simulink model "BirdEyeView_Bilinear_V1"  (R2022a)
settings: Solver=FixedStepDiscrete  StartTime=0.0  StopTime=Ts_480p*4  RelTol=1e-3
InitFcn:
  | Ts = 1e-3;
  | Ts_240p = 402*324*Ts;
  | Ts_480p = 525*800*Ts;
  | %global lut;
  | %temp = load('lut_rc_c.mat');
  | %lut = temp.lut_rc_c;
undefined symbols (not defined in the file or in its folder): gray, Rec, SDTV
libraries: hdlsllib x13, visionhdlio x2, visionhdlconversions x1, dspvision x1
settings Model: DataTypeOverride=Off  ModifiedByFormat=4mbilal@gmail.com  Creator=The MathWorks, Inc.  LastModifiedBy=4mbilal@gmail.com
settings SolverCC: AlgebraicLoopSolver=TrustRegion
settings DataIOCC: LimitDataPoints=on  SaveFormat=Array  SaveOutput=off  SaveTime=off  ReturnWorkspaceOutputs=off
settings OptimizationCC: BlockReduction=off  ConditionallyExecuteInputs=off  DefaultParameterBehavior=Inlined  LifeSpan=inf
settings DebuggingCC: AlgebraicLoopMsg=error  SolverPrmCheckMsg=warning  SingleTaskRateTransMsg=error  ParameterPrecisionLossMsg=none  UnconnectedInputMsg=warning  UnconnectedOutputMsg=warning  UnconnectedLineMsg=warning  AllowSymbolicDim=off  SFUnexpectedBacktrackingDiag=warning  SFNoUnconditionalDefaultTransitionDiag=warning  SFExecutionAtInitializationDiag=none  SFMachineParentedDataDiag=warning  IntegerSaturationMsg=none  ArithmeticOperatorsInVariantConditions=warning
settings HardwareCC: ProdBitPerPointer=32  ProdBitPerSizeT=32  ProdBitPerPtrDiffT=32  ProdLargestAtomicFloat=None  ProdIntDivRoundTo=Undefined  ProdEndianess=Unspecified  ProdWordSize=32  ProdHWDeviceType=ASIC/FPGA->ASIC/FPGA  ProdEqTarget=off
settings ModelReferenceCC: PropagateSignalLabelsOutOfModel=off
settings SFSimCC: SimUseLocalCustomCode=off  CustomCodeUndefinedFunction=UseInterfaceOnly
settings RTWCC: RTWUseLocalCustomCode=off
settings CodeAppCC: StateflowObjectComments=on
settings GRTTargetCC: TargetLangStandard=C89/C90 (ANSI)
settings ConfigComp: CovMetricSettings=dw  CovSaveCumulativeToWorkspaceVar=on  CovSaveSingleToWorkspaceVar=on  CovExternalEMLEnable=off  CovSFcnEnable=off

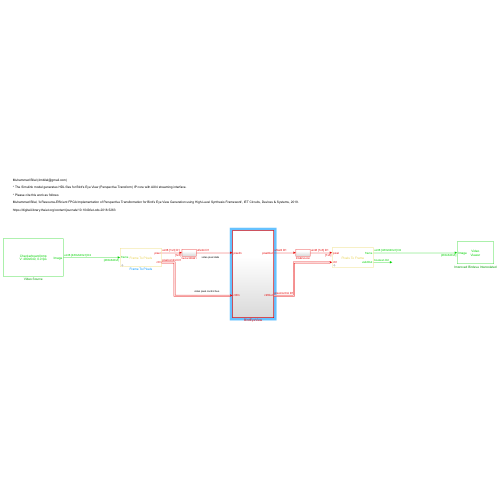
[thumbnail: Simulink's stored preview of the top-level diagram]
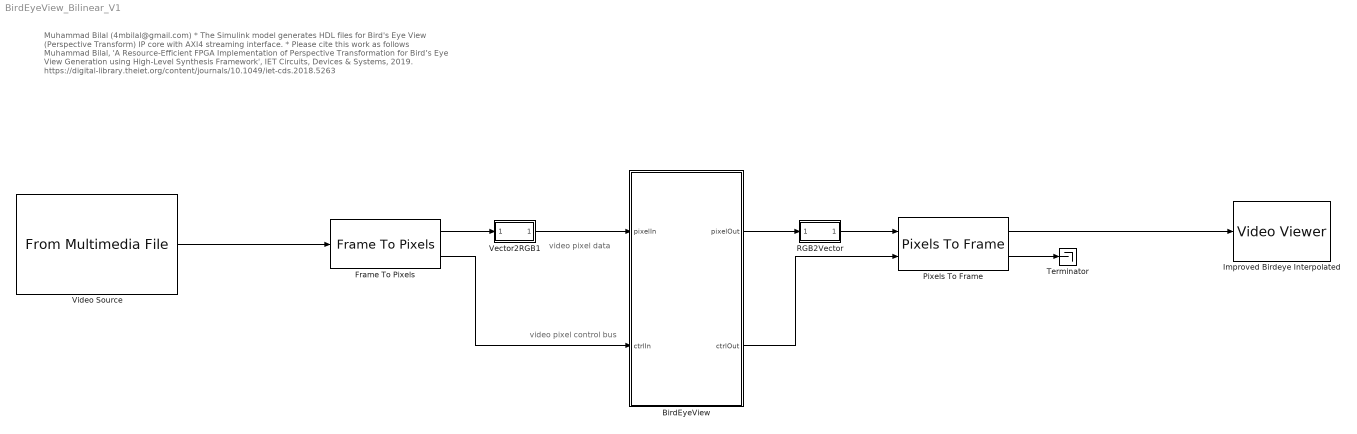
== system BirdEyeView_Bilinear_V1 ==
  note: Muhammad Bilal (4mbilal@gmail.com)
      |
      | * The Simulink model generates HDL files for Bird's Eye View (Perspective Transform) IP core with AXI4 streaming interface.
      |
      | * Please cite this work as follows
      |
      | Muhammad Bilal, 'A Resource-Efficient FPGA Implementation of Perspective Transformation for Bird’s Eye View Generation using High-Level Synthesis Framework', IET Circuits, Devices & Systems, 2019.
      |
      | https://digital-library.theiet.org/content/journals/10.1049/iet-cds.2018.5263
  note: video pixel data
  note: video pixel control bus
  BirdEyeView : Subsystem  TreatAsAtomicUnit=on
  Frame To Pixels : visionhdlio/Frame To Pixels  NumComponents=3  NumPixels=1  VideoFormat=480p  ActivePixelsPerLine=640  ActiveVideoLines=480  TotalPixelsPerLine=800  TotalVideoLines=525  StartingActiveLine=36  FrontPorch=16  SampleTime=0  VideoFormatCache=480p  ActivePixelsPerLineCache=32  ActiveVideoLinesCache=18  TotalPixelsPerLineCache=42  TotalVideoLinesCache=28  StartingActiveLineCache=6  FrontPorchCache=5
      settings: SourceProductBaseCode=VT
  Improved Birdeye Interpolated : VideoViewer  colormapValue=gray(256)  FigPos=[601 632.4 660.8 447.2]
  Pixels To Frame : visionhdlio/Pixels To Frame  NumComponents=3  NumPixels=1  VideoFormat=480p  ActivePixelsPerLine=640  ActiveVideoLines=480  TotalPixelsPerLine=800  TotalVideoLines=525  VideoFormatCache=480p  ActivePixelsPerLineCache=32  ActiveVideoLinesCache=18  TotalPixelsPerLineCache=42  TotalVideoLinesCache=28
      settings: SourceProductBaseCode=VT
  RGB2Vector : Subsystem
  Terminator : Terminator
  Vector2RGB1 : Subsystem
  Video Source : dspvision/From Multimedia File  inputFilename=D:\Zedboard\custom_ip_cores\Mathworks\BirdsEyeView\Checkerboard.bmp  readRange=[1 Inf]  loop=on  numPlays=inf  outputStreams=Video only  videoDataType=uint8  audioDataType=int16  inheritSampleTime=off  userDefinedSampleTime=Ts_480p  noAudioOutput=off  isIntensityVideo=off  fourcc=RGB  colorVideoFormat=One multidimensional signal  outputEOF=off  dataOrg=Column-major  audioFrameSize=1024  computeAudioFrameSize=off  outSamplingMode=Sample based
  wires:
  Pixels To Frame/2 -> Terminator/1
  Vector2RGB1/1(RGB) -> BirdEyeView/1(pixelIn)
  BirdEyeView/1(pixelOut) -> RGB2Vector/1(RGB)
  Frame To Pixels/1 -> Vector2RGB1/1(RGBVector)
  BirdEyeView/2(ctrlOut) -> Pixels To Frame/2
  Frame To Pixels/2 -> BirdEyeView/2(ctrlIn)
  RGB2Vector/1(RGBVector) -> Pixels To Frame/1
  Pixels To Frame/1 -> Improved Birdeye Interpolated/1
  Video Source/1 -> Frame To Pixels/1

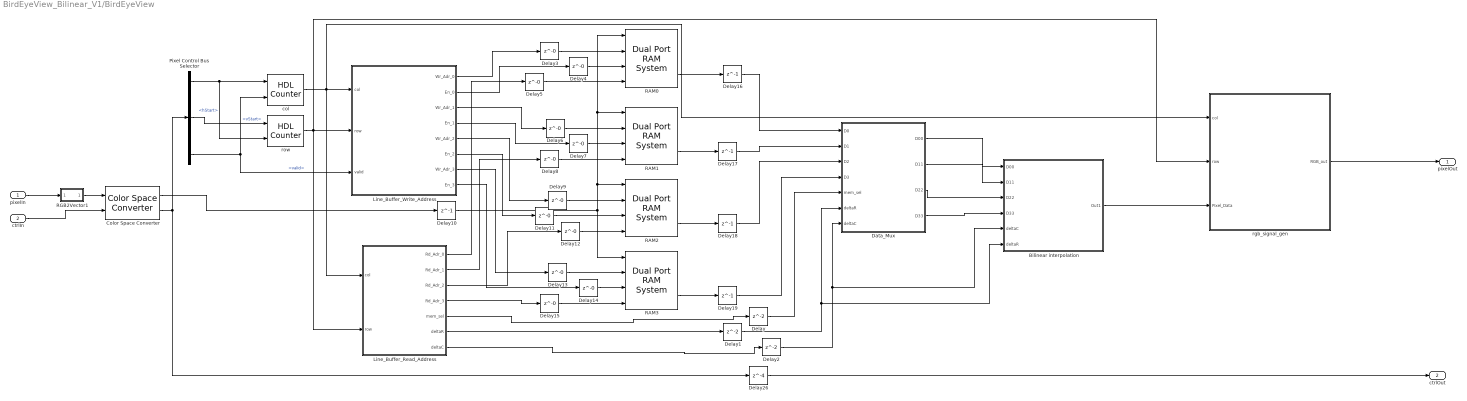
== system BirdEyeView_Bilinear_V1/BirdEyeView ==
  pixelIn : Inport
  ctrlIn : Inport  Port=2
  Bilinear interpolation : Subsystem
  Color Space Converter : visionhdlconversions/Color Space Converter  Conversion=RGB to intensity  ConversionStandard=Rec. 601 (SDTV)  ScanningStandard=1250/50/2:1  SimulateUsing=Code generation
      settings: SourceProductBaseCode=VT
  Data_Mux : MATLAB Function  TreatAsAtomicUnit=on
  Delay : Delay  InitialCondition=0
  Delay1 : Delay  InitialCondition=0
  Delay{10,16..19} (5 alike) : Delay  DelayLength=1  InitialCondition=0
  Delay{3..9,11..15} (12 alike) : Delay  DelayLength=0  InitialCondition=0
  Delay2 : Delay  InitialCondition=0
  Delay26 : Delay  DelayLength=4  InitialCondition=0
  Line_Buffer_Read_Address : MATLAB Function  TreatAsAtomicUnit=on
  Line_Buffer_Write_Address : MATLAB Function  TreatAsAtomicUnit=on
  Pixel Control Bus Selector : BusSelector  OutputSignals=hStart,hEnd,vStart,vEnd,valid
  RAM{0..3} (4 alike) : hdlsllib/HDL RAMs/Dual Port RAM System  RAMType=Dual port  WriteOutputValue=New data  RAMInitialValue=0  SimulateUsing=Code generation
      settings: SourceProductBaseCode=SL
  RGB2Vector1 : Subsystem
  col : hdlsllib/Sources/HDL Counter  CountType=Count limited  CountInit=0  CountStep=1  CountMax=638  CountFromType=Initial value  CountFrom=0  CountResetPort=on  CountLoadPort=off  CountEnbPort=on  CountDirPort=off  CountHitOutputPort=off  CountDataType=Unsigned  CountWordLen=10  CountFracLen=0  CountSampTime=1
  rgb_signal_gen : MATLAB Function  TreatAsAtomicUnit=on
  row : hdlsllib/Sources/HDL Counter  CountType=Count limited  CountInit=0  CountStep=1  CountMax=638  CountFromType=Initial value  CountFrom=0  CountResetPort=on  CountLoadPort=off  CountEnbPort=on  CountDirPort=off  CountHitOutputPort=off  CountDataType=Unsigned  CountWordLen=10  CountFracLen=0  CountSampTime=1
  pixelOut : Outport  VectorParamsAs1DForOutWhenUnconnected=off
  ctrlOut : Outport  Port=2  VectorParamsAs1DForOutWhenUnconnected=off
  wires:
  ctrlIn/1 -> Color Space Converter/2
  pixelIn/1 -> RGB2Vector1/1(RGB)
  RGB2Vector1/1(RGBVector) -> Color Space Converter/1
  rgb_signal_gen/1(RGB_out) -> pixelOut/1
  Color Space Converter/2 -> Delay26/1, Pixel Control Bus Selector/1
  Pixel Control Bus Selector/1 -> row/2, col/1  "<hStart>"
  col/1 -> Line_Buffer_Read_Address/1(col), Line_Buffer_Write_Address/1(col), rgb_signal_gen/1(col)
  Pixel Control Bus Selector/5 -> Line_Buffer_Write_Address/3(valid), col/2  "<valid>"
  Pixel Control Bus Selector/3 -> row/1  "<vStart>"
  row/1 -> Line_Buffer_Read_Address/2(row), Line_Buffer_Write_Address/2(row), rgb_signal_gen/2(row)
  Color Space Converter/1 -> Delay10/1
  Line_Buffer_Write_Address/1(Wr_Adr_0) -> Delay3/1
  Line_Buffer_Write_Address/2(En_0) -> Delay4/1
  Line_Buffer_Write_Address/3(Wr_Adr_1) -> Delay6/1
  Line_Buffer_Write_Address/4(En_1) -> Delay7/1
  Line_Buffer_Write_Address/5(Wr_Adr_2) -> Delay9/1
  Line_Buffer_Write_Address/6(En_2) -> Delay11/1
  Line_Buffer_Write_Address/7(Wr_Adr_3) -> Delay13/1
  Line_Buffer_Write_Address/8(En_3) -> Delay14/1
  Line_Buffer_Read_Address/1(Rd_Adr_0) -> Delay5/1
  Line_Buffer_Read_Address/2(Rd_Adr_1) -> Delay8/1
  Line_Buffer_Read_Address/3(Rd_Adr_2) -> Delay12/1
  Line_Buffer_Read_Address/4(Rd_Adr_3) -> Delay15/1
  RAM0/2 -> Delay16/1
  RAM1/2 -> Delay17/1
  RAM2/2 -> Delay18/1
  RAM3/2 -> Delay19/1
  Line_Buffer_Read_Address/5(mem_sel) -> Delay/1
  Line_Buffer_Read_Address/6(deltaR) -> Delay1/1
  Line_Buffer_Read_Address/7(deltaC) -> Delay2/1
  Delay/1 -> Data_Mux/5(mem_sel)
  Delay1/1 -> Data_Mux/6(deltaR), Bilinear interpolation/6(deltaR)
  Delay2/1 -> Data_Mux/7(deltaC), Bilinear interpolation/5(deltaC)
  Delay3/1 -> RAM0/2
  Delay4/1 -> RAM0/3
  Delay5/1 -> RAM0/4
  Delay6/1 -> RAM1/2
  Delay7/1 -> RAM1/3
  Delay8/1 -> RAM1/4
  Delay9/1 -> RAM2/2
  Delay10/1 -> RAM0/1, RAM1/1, RAM2/1, RAM3/1
  Delay11/1 -> RAM2/3
  Delay12/1 -> RAM2/4
  Delay13/1 -> RAM3/2
  Delay14/1 -> RAM3/3
  Delay15/1 -> RAM3/4
  Delay16/1 -> Data_Mux/1(D0)
  Delay17/1 -> Data_Mux/2(D1)
  Delay18/1 -> Data_Mux/3(D2)
  Delay19/1 -> Data_Mux/4(D3)
  Delay26/1 -> ctrlOut/1
  Data_Mux/1(D00) -> Bilinear interpolation/1(D00)
  Data_Mux/2(D11) -> Bilinear interpolation/2(D11)
  Data_Mux/3(D22) -> Bilinear interpolation/3(D22)
  Data_Mux/4(D33) -> Bilinear interpolation/4(D33)
  Bilinear interpolation/1(Out1) -> rgb_signal_gen/3(Pixel_Data)

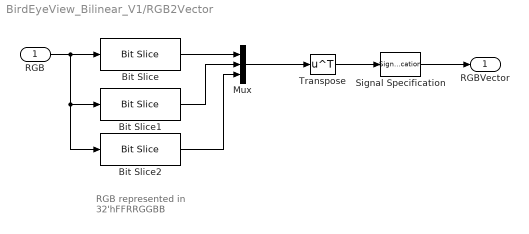
== system BirdEyeView_Bilinear_V1/RGB2Vector ==
  note: RGB represented in
      | 32'hFFRRGGBB
  RGB : Inport
  Bit Slice : hdlsllib/Logic and Bit Operations/Bit Slice  lidx=23  ridx=16
      settings: SourceProductBaseCode=SL
  Bit Slice1 : hdlsllib/Logic and Bit Operations/Bit Slice  lidx=15  ridx=8
      settings: SourceProductBaseCode=SL
  Bit Slice2 : hdlsllib/Logic and Bit Operations/Bit Slice  lidx=7  ridx=0
      settings: SourceProductBaseCode=SL
  Mux : Mux  Inputs=3
  Signal Specification : SignalSpecification
  Transpose : Math  Operator=transpose  SignedPower=on
  RGBVector : Outport  VectorParamsAs1DForOutWhenUnconnected=off
  wires:
  Mux/1 -> Transpose/1
  Bit Slice/1 -> Mux/1
  Bit Slice2/1 -> Mux/3
  Bit Slice1/1 -> Mux/2
  RGB/1 -> Bit Slice2/1, Bit Slice1/1, Bit Slice/1
  Transpose/1 -> Signal Specification/1
  Signal Specification/1 -> RGBVector/1

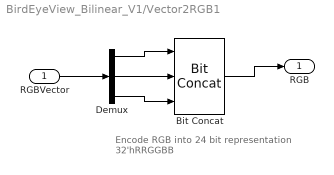
== system BirdEyeView_Bilinear_V1/Vector2RGB1 ==
  note: Encode RGB into 24 bit representation
      | 32'hRRGGBB
  RGBVector : Inport
  Bit Concat : hdlsllib/Logic and Bit Operations/Bit Concat  numInputs=3
  Demux : Demux  Outputs=3
  RGB : Outport  VectorParamsAs1DForOutWhenUnconnected=off
  wires:
  Bit Concat/1 -> RGB/1
  RGBVector/1 -> Demux/1
  Demux/1 -> Bit Concat/1
  Demux/2 -> Bit Concat/2
  Demux/3 -> Bit Concat/3

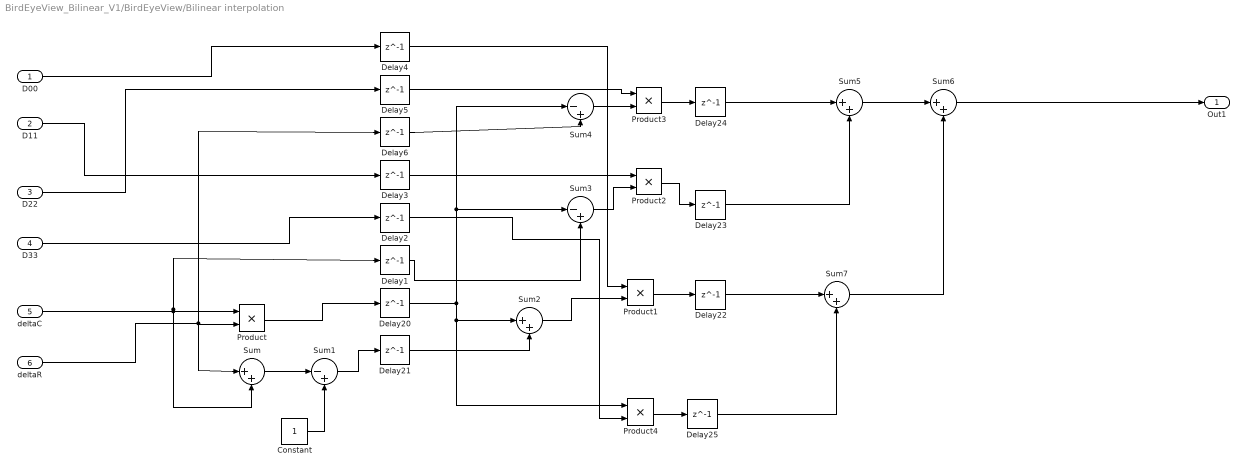
== system BirdEyeView_Bilinear_V1/BirdEyeView/Bilinear interpolation ==
  D00 : Inport
  D11 : Inport  Port=2
  D22 : Inport  Port=3
  D33 : Inport  Port=4
  deltaC : Inport  Port=5
  deltaR : Inport  Port=6
  Constant : Constant  OutDataTypeStr=boolean
  Delay{1..6,20..25} (12 alike) : Delay  DelayLength=1  InitialCondition=0
  Product{,1..4} (5 alike) : Product
  Sum{,2,5..7} (5 alike) : Sum  Inputs=|++
  Sum1 : Sum  Inputs=|-+
  Sum3 : Sum  Inputs=|-+
  Sum4 : Sum  Inputs=|-+
  Out1 : Outport  VectorParamsAs1DForOutWhenUnconnected=off
  wires:
  D11/1 -> Delay3/1
  Product1/1 -> Delay22/1
  Sum4/1 -> Product3/2
  Product3/1 -> Delay24/1
  Delay21/1 -> Sum2/2
  D22/1 -> Delay5/1
  Delay20/1 -> Product4/1, Sum2/1, Sum4/1, Sum3/1
  deltaC/1 -> Delay1/1, Product/1, Sum/2
  deltaR/1 -> Delay6/1, Sum/1, Product/2
  Sum2/1 -> Product1/2
  Sum6/1 -> Out1/1
  Constant/1 -> Sum1/2
  Product/1 -> Delay20/1
  Sum3/1 -> Product2/2
  Delay23/1 -> Sum5/2
  Sum5/1 -> Sum6/1
  D00/1 -> Delay4/1
  Sum1/1 -> Delay21/1
  Product2/1 -> Delay23/1
  Sum/1 -> Sum1/1
  Delay22/1 -> Sum7/1
  Sum7/1 -> Sum6/2
  Delay25/1 -> Sum7/2
  D33/1 -> Delay2/1
  Delay24/1 -> Sum5/1
  Product4/1 -> Delay25/1
  Delay1/1 -> Sum3/2
  Delay2/1 -> Product4/2
  Delay3/1 -> Product2/1
  Delay4/1 -> Product1/1
  Delay5/1 -> Product3/1
  Delay6/1 -> Sum4/2

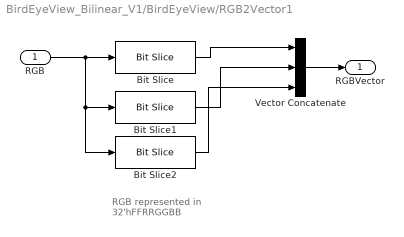
== system BirdEyeView_Bilinear_V1/BirdEyeView/RGB2Vector1 ==
  note: RGB represented in
      | 32'hFFRRGGBB
  RGB : Inport
  Bit Slice : hdlsllib/Logic and Bit Operations/Bit Slice  lidx=23  ridx=16
      settings: SourceProductBaseCode=SL
  Bit Slice1 : hdlsllib/Logic and Bit Operations/Bit Slice  lidx=15  ridx=8
      settings: SourceProductBaseCode=SL
  Bit Slice2 : hdlsllib/Logic and Bit Operations/Bit Slice  lidx=7  ridx=0
      settings: SourceProductBaseCode=SL
  Vector Concatenate : Concatenate  NumInputs=3  Mode=Multidimensional array  ConcatenateDimension=2
  RGBVector : Outport  VectorParamsAs1DForOutWhenUnconnected=off
  wires:
  Bit Slice/1 -> Vector Concatenate/1
  Bit Slice2/1 -> Vector Concatenate/3
  Bit Slice1/1 -> Vector Concatenate/2
  RGB/1 -> Bit Slice2/1, Bit Slice1/1, Bit Slice/1
  Vector Concatenate/1 -> RGBVector/1

== matlab function BirdEyeView_Bilinear_V1/BirdEyeView/Line_Buffer_Read_Address ==
  data: col input; Rd_Adr_0 output; row input; Rd_Adr_1 output; Rd_Adr_2 output; Rd_Adr_3 output; mem_sel output; deltaR output; deltaC output
function [Rd_Adr_0,Rd_Adr_1,Rd_Adr_2,Rd_Adr_3,mem_sel,deltaR, deltaC]  = rd_adr_gen(col,row)
% r_in = double(r);
% c_in = double(c);

% col_adr = (216.3 - 0.06823*r_in + 0.3218*c_in - 0.000236*r_in^2 + 0.0002136*r_in*c_in + 0.0000007421*r_in^2*c_in);
% row_adr = (196.8 + 0.01674*r_in + 5.779e-05*r_in^2);


% Fixed-point 24-bit implementation
r_in = fi(row,0,9,0);
c_in = fi(col,0,10,0);

% c1 = fi(216.3);
c1 = fi(215.8); %-0.5 for flooring
c2 = fi(-0.06823);
c3 = fi(0.3218);
c4 = fi(-0.000236);
c5 = fi(0.0002136);
c6 = fi(0.0000007421);
col_adr = (c1 + c2*r_in + c3*c_in + c4*r_in^2 + c5*r_in*c_in + c6*r_in^2*c_in);
c7 = fi(0.06125);
% col_adr = c_in*c7;

% r1 = fi(196.8);
r1 = fi(0.8);
% r1 = fi(0.3);%-0.5 for flooring
r2 = fi(0.01674);
r3 = fi(5.779e-05);
row_adr = (r1 + r2*r_in + r3*r_in^2);
r4 = fi(0.06125);
% row_adr = r_in*r4;

row_adr_fi = fi(row_adr, 0, 9, 0);
col_adr_fi = fi(col_adr, 0, 10, 0);

deltaR = row_adr - row_adr_fi;
deltaC = col_adr - col_adr_fi;

mem_sel = bitconcat(bitget(row_adr_fi,1),bitget(col_adr_fi,1));
Base_Adr = row_adr_fi*fi(160) + col_adr_fi*fi(0.5);

switch(mem_sel)
    case {0}
            A0r = fi(0,1,2,0);
            A0c = fi(0,1,2,0);
            A1r = fi(0,1,2,0);
            A1c = fi(0,1,2,0);
            A2r = fi(0,1,2,0);
            A2c = fi(0,1,2,0);
            A3r = fi(0,1,2,0);
            A3c = fi(0,1,2,0);
    case {1}
            A0r = fi(0,1,2,0);
            A0c = fi(1,1,2,0);
            A1r = fi(0,1,2,0);
            A1c = fi(-1,1,2,0);
            A2r = fi(0,1,2,0);
            A2c = fi(1,1,2,0);
            A3r = fi(0,1,2,0);
            A3c = fi(-1,1,2,0);
    case {2}
            A0r = fi(1,1,2,0);
            A0c = fi(0,1,2,0);
            A1r = fi(1,1,2,0);
            A1c = fi(0,1,2,0);
            A2r = fi(-1,1,2,0);
            A2c = fi(0,1,2,0);
            A3r = fi(-1,1,2,0);
            A3c = fi(0,1,2,0);
    case {3}
            A0r = fi(1,1,2,0);
            A0c = fi(1,1,2,0);
            A1r = fi(1,1,2,0);
            A1c = fi(-1,1,2,0);
            A2r = fi(-1,1,2,0);
            A2c = fi(1,1,2,0);
            A3r = fi(-1,1,2,0);
            A3c = fi(-1,1,2,0);
    otherwise
            A0r = fi(0,1,2,0);
            A0c = fi(0,1,2,0);
            A1r = fi(0,1,2,0);
            A1c = fi(0,1,2,0);
            A2r = fi(0,1,2,0);
            A2c = fi(0,1,2,0);
            A3r = fi(0,1,2,0);
            A3c = fi(0,1,2,0);
end 

A0 = A0r*fi(160) + A0c*fi(0.5);
A1 = A1r*fi(160) + A1c*fi(0.5);
A2 = A2r*fi(160) + A2c*fi(0.5);
A3 = A3r*fi(160) + A3c*fi(0.5);

Rd_Adr_0 = fi(Base_Adr + A0,0,12,0);
Rd_Adr_1 = fi(Base_Adr + A1,0,12,0);
Rd_Adr_2 = fi(Base_Adr + A2,0,12,0);
Rd_Adr_3 = fi(Base_Adr + A3,0,12,0);

%Memory Size = 25*160=4000(=2^12)

== matlab function BirdEyeView_Bilinear_V1/BirdEyeView/rgb_signal_gen ==
  data: col input; row input; Pixel_Data input; RGB_out output
function RGB_out  = rgb_signal_gen(col,row,Pixel_Data)

in_d = (Pixel_Data);%Double precision format
% if(row<196)
%     in_d = 0;
% elseif(row>430)
%     in_d = 0;
% end
% if(col<50)
%     in_d = 0;
% elseif(col>590)
%     in_d = 0;
% end

R = fi(in_d, 0, 8, 0);%convert to fixed-point 8-bit signal
G = fi(in_d, 0, 8, 0);
B = fi(in_d, 0, 8, 0);
A = fi(255, 0, 8, 0);

% RGB_out = bitconcat(A,R,G,B);%32-bit output signal

RGB_out = bitconcat(R,G,B);%32-bit output signal

== matlab function BirdEyeView_Bilinear_V1/BirdEyeView/Line_Buffer_Write_Address ==
  data: col input; Wr_Adr_0 output; En_0 output; row input; Wr_Adr_1 output; En_1 output; Wr_Adr_2 output; En_2 output; Wr_Adr_3 output; En_3 output; valid input
function [Wr_Adr_0,En_0,Wr_Adr_1,En_1,Wr_Adr_2,En_2,Wr_Adr_3,En_3]  = Lin_Buf_Wr_Adr(col,row,valid)

% row_adr = fi(row,0,9,0);
% col_adr = fi(col,0,10,0);
row = double(row);
col = double(col);


%The following code ensures that row is always within the range [0 24],
%Row 24 is the dump for unwanted rows <196 and >219. 
if((row<196)|(row>219))
    row = 24;
    Dump = 0;
else
    row = row - 196;
    Dump = 1;
end
% Dump = 1;

row_adr = fi(row,0,9,0);
col_adr = fi(col,0,10,0);
Dump_fi = fi(Dump,0,1,0);

full_adr_0 = row_adr*fi(160) + col_adr*fi(0.5);
full_adr_1 = full_adr_0 - 0.5;
full_adr_2 = full_adr_0 - 160;
full_adr_3 = full_adr_0 - 160.5;
% full_adr_1 = row_adr*fi(160) + (col_adr-1)*fi(0.5);
% full_adr_2 = (row_adr-1)*fi(160) + col_adr*fi(0.5);
% full_adr_3 = (row_adr-1)*fi(160) + (col_adr-1)*fi(0.5);

%Memory Size = 25*160=4000(=2^12)
Wr_Adr_0 = fi(full_adr_0, 0, 12, 0);
Wr_Adr_1 = fi(full_adr_1, 0, 12, 0);
Wr_Adr_2 = fi(full_adr_2, 0, 12, 0);
Wr_Adr_3 = fi(full_adr_3, 0, 12, 0);

En_0 = (~double(bitget(row_adr,1)))&(~double(bitget(col_adr,1)))&valid&Dump_fi;
En_1 = (~double(bitget(row_adr,1)))&(double(bitget(col_adr,1)))&valid&Dump_fi;
En_2 = (double(bitget(row_adr,1)))&(~double(bitget(col_adr,1)))&valid;
En_3 = (double(bitget(row_adr,1)))&(double(bitget(col_adr,1)))&valid;

== matlab function BirdEyeView_Bilinear_V1/BirdEyeView/Data_Mux ==
  data: D0 input; D1 input; D2 input; D3 input; mem_sel input; deltaR input; deltaC input; D00 output; D11 output; D22 output; D33 output
function [D00, D11, D22, D33] = Rd_Data_Mux(D0,D1,D2,D3,mem_sel,deltaR, deltaC)

switch(mem_sel)
    case {0}
            D00 = D0;
            D11 = D1;
            D22 = D2;
            D33 = D3;
    case {1}
            D00 = D1;
            D11 = D0;
            D22 = D3;
            D33 = D2;
    case {2}
            D00 = D2;
            D11 = D3;
            D22 = D0;
            D33 = D1;
    case {3}
            D00 = D3;
            D11 = D2;
            D22 = D1;
            D33 = D0;
    otherwise
            D00 = uint8(0);
            D11 = uint8(0);
            D22 = uint8(0);
            D33 = uint8(0);
end 

% deltaRC_3 = deltaR*deltaC;
% deltaRC_2 = deltaR - deltaRC_3;
% deltaRC_1 = deltaC - deltaRC_3;
% deltaRC_0 = 1-deltaR-deltaC+deltaRC_3;
% 
% Data_interp = D00*deltaRC_0 + D11*deltaRC_1 +D22*deltaRC_2 +D33*deltaRC_3;
% Data_interp = D11*(1-deltaR) + D33*(deltaR);
% Data_interp = D00*(1-deltaR) + D22*(deltaR);
% Data_interp = D00*(1-deltaC) + D11*(deltaC);
% Data_interp = D22*(1-deltaC) + D33*(deltaC);
% Data_interp = D00;
% Data_Out = fi(Data_interp,0,8,0);
